simulink model "Problem2_2"  (R2018a)
settings: Solver=VariableStepAuto  StartTime=0.0  StopTime=10.0  RelTol=1e-3
settings Model: Creator=NIMA  LastModifiedBy=NIMA

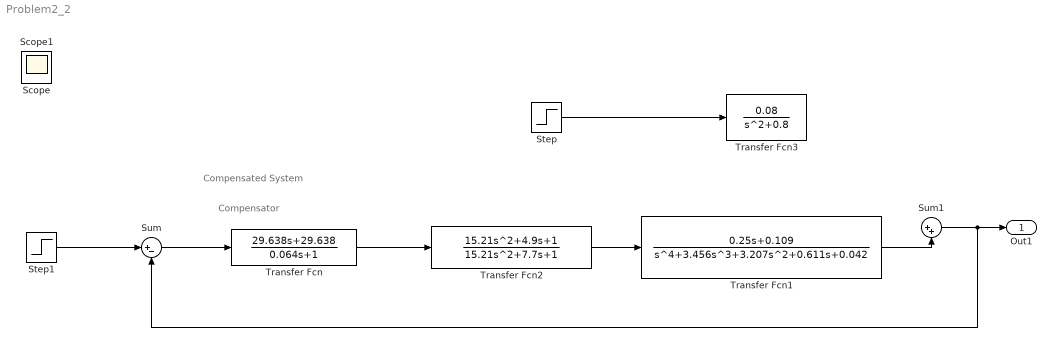
== system Problem2_2 ==
  note: Compensated System
  note: Compensator
  Step : Step  SampleTime=0
  Step1 : Step  SampleTime=0
  Sum : Sum  Inputs=|+-
  Sum1 : Sum  Inputs=|++
  Transfer Fcn : TransferFcn  Numerator=[29.638 29.638]  Denominator=[0.064 1]
  Transfer Fcn1 : TransferFcn  Numerator=[0.25 0.109]  Denominator=[1 3.456 3.207 0.611 0.042]
  Transfer Fcn2 : TransferFcn  Numerator=[15.21 4.9 1]  Denominator=[15.21 7.7 1]
  Transfer Fcn3 : TransferFcn  Numerator=[0.08]  Denominator=[1 0 0.8]
  Out1 : Outport
  Scope : Scope
  Scope1 : Scope
  wires:
  Step1/1 -> Sum/1
  Transfer Fcn/1 -> Transfer Fcn2/1
  Sum/1 -> Transfer Fcn/1
  Transfer Fcn2/1 -> Transfer Fcn1/1
  Transfer Fcn1/1 -> Sum1/2
  Step/1 -> Transfer Fcn3/1
  Sum1/1 -> Sum/2, Out1/1
